simulink model "flight1"  (R2016a)
settings: Solver=VariableStepAuto  StartTime=0.0  StopTime=10.0  RelTol=1e-3
settings Model: Creator=ganam  LastModifiedBy=ganam

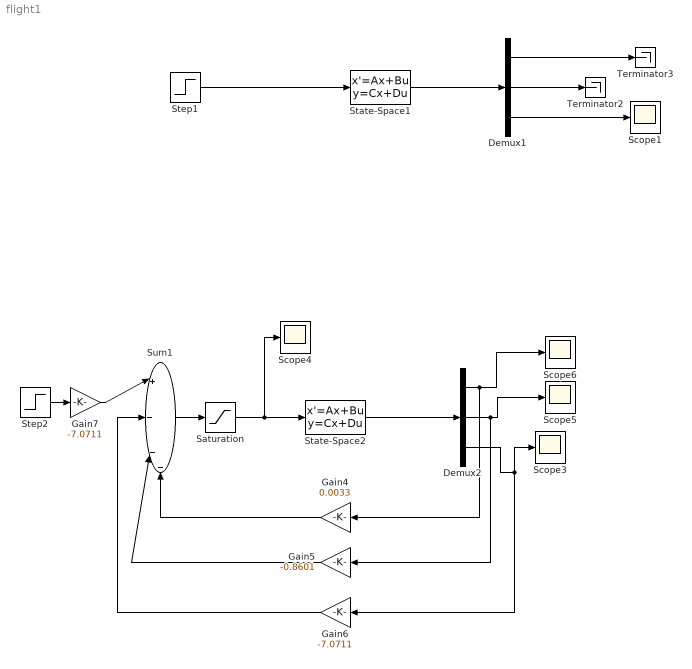
== system flight1 ==
  Demux1 : Demux  Outputs=3
  Demux2 : Demux  Outputs=3
  Gain4 : Gain  Gain=0.0033
  Gain5 : Gain  Gain=-0.8601
  Gain6 : Gain  Gain=-7.0711
  Gain7 : Gain  Gain=-7.0711
  Saturation : Saturate  UpperLimit=.5  LowerLimit=-.5
  Scope{1,3..6} (5 alike) : Scope
  State-Space1 : StateSpace  A=[-.452 70 0 ; -.006 -.317 0 ; 0 1 0]  B=[-2.03 ; -1.46 ; 0]  C=eye(3)  D=[0;0;0]  X0=0  ContinuousStateAttributes={'w','q','pitch'}
  State-Space2 : StateSpace  A=[-1.33 237.1 0 ; -.051 -1.09 0 ; 0 1 0 ]  B=[-22.4 ; -14.5 ; 0]  C=eye(3)  D=[0;0;0]  X0=0  ContinuousStateAttributes={'w','q','pitch'}
  Step1 : Step  Time=0  After=.2  SampleTime=0
  Step2 : Step  Time=0  After=.2  SampleTime=0
  Sum1 : Sum  Inputs=|+---
  Terminator2 : Terminator
  Terminator3 : Terminator
  wires:
  State-Space1/1 -> Demux1/1
  Demux1/3 -> Scope1/1
  Demux1/1 -> Terminator3/1
  Demux1/2 -> Terminator2/1
  Step1/1 -> State-Space1/1
  State-Space2/1 -> Demux2/1
  Demux2/3 -> Gain6/1, Scope3/1
  Demux2/1 -> Scope6/1, Gain4/1
  Demux2/2 -> Scope5/1, Gain5/1
  Sum1/1 -> Saturation/1
  Gain4/1 -> Sum1/4
  Gain5/1 -> Sum1/3
  Gain6/1 -> Sum1/2
  Step2/1 -> Gain7/1
  Gain7/1 -> Sum1/1
  Saturation/1 -> Scope4/1, State-Space2/1
